simulink model "simul"  (R2014b)
settings: Solver=ode3  StartTime=0.0  StopTime=T  FixedStep=dt  RelTol=1e-3
values from neighbouring files (symbols this model uses):
  dt = T/samples    (= 0.00732421875)    [play_simul.m]
  samples = 2^10    (= 1024)    [LD5script.m]    (also in play_simul.m = 4096)
  T = 5    [LD5script.m]    (also in play_simul.m = 30)
  tau = 1    [play_simul.m]
libraries: dsparch4 x2, dspstat3 x2, dspxfrm3 x1, commnoisgen2 x1
settings Model: Creator=Armands  LastModifiedBy=Armands

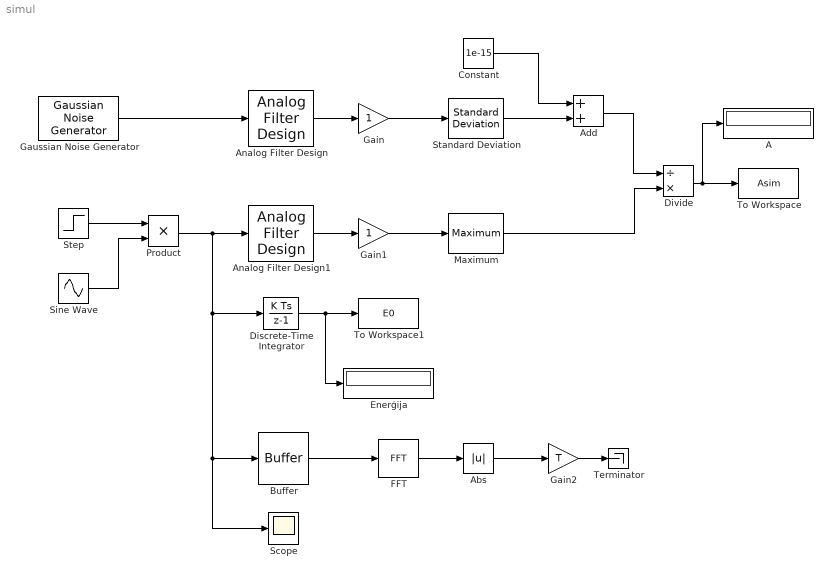
== system simul ==
  A : Display
  Abs : Abs
  Add : Sum
  Analog Filter Design : dsparch4/Analog Filter Design  method=Butterworth  filttype=Lowpass  N=1  Wlo=2.63632  Whi=80  Rp=2  Rs=40
  Analog Filter Design1 : dsparch4/Analog Filter Design  method=Butterworth  filttype=Lowpass  N=1  Wlo=2.63632  Whi=80  Rp=2  Rs=40
  Buffer : Buffer  N=samples  TreatMby1Signals=One channel
  Constant : Constant  Value=1e-15  SampleTime=dt
  Discrete-Time Integrator : DiscreteIntegrator  InitialConditionSetting=State (most efficient)  SampleTime=dt
  Divide : Product  Inputs=/*
  Enerģija : Display
  FFT : dspxfrm3/FFT  CompMethod=Table lookup  TableOpt=NEW  TableOptActive=Speed  BitRevOrder=off  InheritFFTLength=off  FFTLength=samples  WrapInput=on  RowConvenienceOn=on  FFTImplementation=Auto  SkipNorm=on  firstCoeffDataTypeStr=Inherit: Same word length as input  firstCoeffLastDataTypeStr=Inherit: Same word length as input  outputMin=[]  outputMax=[]  roundingMode=Floor  overflowMode=off
  Gain : Gain  SampleTime=dt
  Gain1 : Gain  SampleTime=dt
  Gain2 : Gain  Gain=T
  Gaussian Noise Generator : commnoisgen2/Gaussian Noise Generator  m=0  d=sigma2x  s=seed  Ts=dt  frameBased=off  sampPerFrame=1  orient=off  outDataType=double
  Maximum : dspstat3/Maximum  fcn=Running  reset=None  indexBase=One  operateOver=Entire input  Dimension=1  colComp=on  operation=maximum  roiEnable=off  roiType=Rectangles  roiPortion=Entire ROI  roiOutput=Individual statistics for each ROI  roiFlag=off  accumDataTypeStr=Inherit: Same as product output  accumLastDataTypeStr=Inherit: Same as product output  roundingMode=Floor  overflowMode=off
  Product : Product
  Scope : Scope
  Sine Wave : Sin  Frequency=pi/tau  SampleTime=dt
  Standard Deviation : dspstat3/Standard Deviation  run=on  reset_popup=None  directionMode=Each column  dimension=1  treatSBRowAsCol=on  roiEnable=off  roiType=Rectangles  roiPortion=Entire ROI  roiOutput=Individual statistics for each ROI  roiFlag=off
  Step : Step  Time=tau  Before=1  After=0  SampleTime=dt
  Terminator : Terminator
  To Workspace : ToWorkspace  VariableName=Asim  SampleTime=dt
      settings: MaxDataPoints=1  Save2DSignal=2-D array (concatenate along first dimension)
  To Workspace1 : ToWorkspace  VariableName=E0  SampleTime=dt
      settings: MaxDataPoints=1  Save2DSignal=2-D array (concatenate along first dimension)
  wires:
  Gaussian Noise Generator/1 -> Analog Filter Design/1
  Analog Filter Design/1 -> Gain/1
  Analog Filter Design1/1 -> Gain1/1
  Gain/1 -> Standard Deviation/1
  Constant/1 -> Add/1
  Standard Deviation/1 -> Add/2
  Gain1/1 -> Maximum/1
  Maximum/1 -> Divide/2
  Divide/1 -> A/1, To Workspace/1
  Add/1 -> Divide/1
  Discrete-Time Integrator/1 -> Enerģija/1, To Workspace1/1
  Buffer/1 -> FFT/1
  FFT/1 -> Abs/1
  Abs/1 -> Gain2/1
  Gain2/1 -> Terminator/1
  Product/1 -> Scope/1, Buffer/1, Discrete-Time Integrator/1, Analog Filter Design1/1
  Step/1 -> Product/1
  Sine Wave/1 -> Product/2
